simulink model "hovergames"  (R2020b)
settings: Solver=FixedStepAuto  StartTime=0.0  StopTime=20  RelTol=1e-3  EnableMultiTasking=on
undefined symbols (not defined in the file): hovergames_activesm, hovergames_sm
libraries: px4uORBlib x6, dspstat3 x1
settings Model: SimulationMode=external  ExtModeTrigDuration=10  Creator=fabsmpa  LastModifiedBy=fabsmpa
settings SolverCC: PositivePriorityOrder=on
settings OptimizationCC: EnhancedBackFolding=on  PassReuseOutputArgsAs=Individual arguments  ZeroExternalMemoryAtStartup=off  ZeroInternalMemoryAtStartup=off  MaxStackSize=64  OptimizeBlockOrder=speed  DifferentSizesBufferReuse=on  OptimizationCustomize=off  EfficientTunableParamExpr=on
settings DebuggingCC: ParameterTunabilityLossMsg=error
settings HardwareCC: ProdBitPerPointer=32  ProdBitPerSizeT=32  ProdBitPerPtrDiffT=32  ProdLargestAtomicInteger=Long  ProdLargestAtomicFloat=Double  ProdWordSize=32  ProdLongLongMode=on  ProdHWDeviceType=ARM Compatible->ARM Cortex  TargetLargestAtomicInteger=Long  TargetLargestAtomicFloat=Double  TargetIntDivRoundTo=Zero  TargetEndianess=LittleEndian  TargetHWDeviceType=NXP->Cortex-M4
settings SFSimCC: MATLABDynamicMemAlloc=off  SimTargetLang=C++
settings RTWCC: Description=Embedded Coder  SystemTargetFile=ert.tlc  HardwareBoard=PX4 Pixhawk Series  TLCOptions="-aInlineSetEventsForThisBaseRateFcn=TLC_FALSE -aSuppressMultiTaskScheduler=TLC_FALSE  -aRateBasedStepFcn=0"  GenCodeOnly=on  TemplateMakefile=ert_default_tmf  Toolchain=GNU Tools for ARM Embedded Processors  CodeProfilingInstrumentation=detailed  TargetLang=C++
settings CodeAppCC: ForceParamTrailComments=on  IgnoreCustomStorageClasses=off  OperatorAnnotations=on  SimulinkDataObjDesc=on  SFDataObjDesc=on  InsertBlockDesc=on
settings ERTTargetCC: CodeInterfacePackaging=C++ class  RootIOFormat=Structure reference

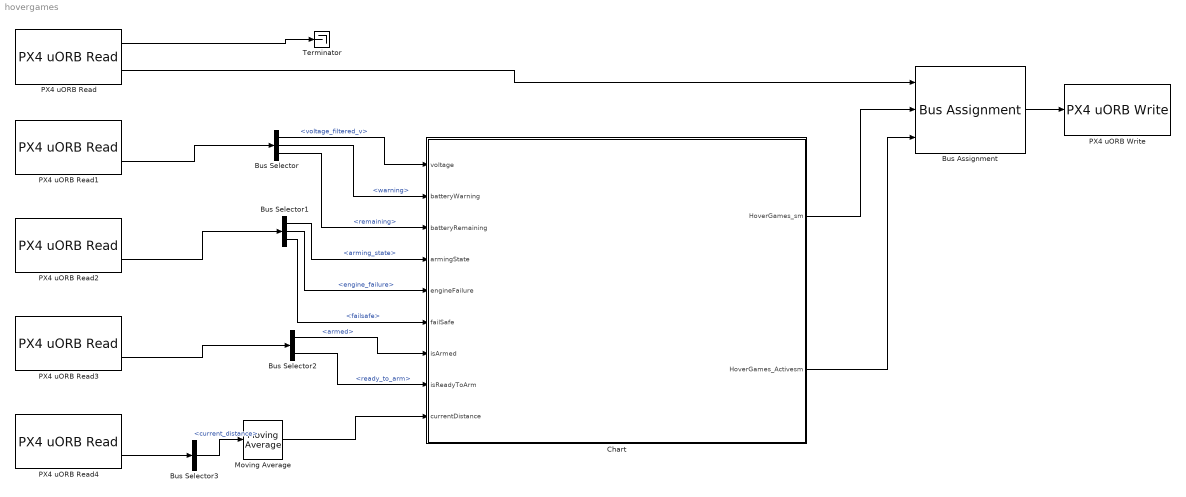
== system hovergames ==
  Bus Assignment : BusAssignment  AssignedSignals=hovergames_sm,hovergames_activesm
  Bus Selector : BusSelector  OutputSignals=voltage_filtered_v,warning,remaining
  Bus Selector1 : BusSelector  OutputSignals=arming_state,engine_failure,failsafe
  Bus Selector2 : BusSelector  OutputSignals=armed,ready_to_arm
  Bus Selector3 : BusSelector  OutputSignals=current_distance
  Chart : Stateflow chart
  Moving Average : dspstat3/Moving Average  Method=Exponential weighting  ForgettingFactorPort=off  SpecifyWindowLength=on  WindowLength=4  ForgettingFactor=0.9  SimulateUsing=Code generation
  PX4 uORB Read : px4uORBlib/PX4 uORB Read  uORBTopic=hovergames  selectInstance=hovergames  SampleTime=0.001  BlockingMode=off  BlockTimeout=1e-3
      settings: SourceProductBaseCode=PX4AUTOPILOTS
  PX4 uORB Read1 : px4uORBlib/PX4 uORB Read  uORBTopic=battery_status  selectInstance=battery_status  SampleTime=0.001  BlockingMode=off  BlockTimeout=1e-3
      settings: SourceProductBaseCode=PX4AUTOPILOTS
  PX4 uORB Read2 : px4uORBlib/PX4 uORB Read  uORBTopic=vehicle_status  selectInstance=vehicle_status  SampleTime=0.001  BlockingMode=off  BlockTimeout=1e-3
      settings: SourceProductBaseCode=PX4AUTOPILOTS
  PX4 uORB Read3 : px4uORBlib/PX4 uORB Read  uORBTopic=actuator_armed  selectInstance=actuator_armed  SampleTime=0.001  BlockingMode=off  BlockTimeout=1e-3
      settings: SourceProductBaseCode=PX4AUTOPILOTS
  PX4 uORB Read4 : px4uORBlib/PX4 uORB Read  uORBTopic=distance_sensor  selectInstance=distance_sensor  SampleTime=0.001  BlockingMode=off  BlockTimeout=1e-3
      settings: SourceProductBaseCode=PX4AUTOPILOTS
  PX4 uORB Write : px4uORBlib/PX4 uORB Write  uORBTopic=hovergames  selectInstance=hovergames  MessageQueueLen=1
      settings: SourceProductBaseCode=PX4AUTOPILOTS
  Terminator : Terminator
  wires:
  PX4 uORB Read/2 -> Bus Assignment/1
  PX4 uORB Read1/2 -> Bus Selector/1
  PX4 uORB Read2/2 -> Bus Selector1/1
  PX4 uORB Read3/2 -> Bus Selector2/1
  PX4 uORB Read4/2 -> Bus Selector3/1
  Bus Selector3/1 -> Moving Average/1  "<current_distance>"
  Bus Selector/1 -> Chart/1(voltage)  "<voltage_filtered_v>"
  Bus Selector/2 -> Chart/2(batteryWarning)  "<warning>"
  Bus Selector/3 -> Chart/3(batteryRemaining)  "<remaining>"
  Bus Selector1/1 -> Chart/4(armingState)  "<arming_state>"
  Bus Selector1/2 -> Chart/5(engineFailure)  "<engine_failure>"
  Bus Selector1/3 -> Chart/6(failSafe)  "<failsafe>"
  Bus Selector2/1 -> Chart/7(isArmed)  "<armed>"
  Bus Selector2/2 -> Chart/8(isReadyToArm)  "<ready_to_arm>"
  Moving Average/1 -> Chart/9(currentDistance)
  Chart/1(HoverGames_sm) -> Bus Assignment/2
  Chart/2(HoverGames_Activesm) -> Bus Assignment/3
  Bus Assignment/1 -> PX4 uORB Write/1
  PX4 uORB Read/1 -> Terminator/1

== stateflow chart hovergames/Chart ==
  state Faulted
    entry:
    HoverGames_sm = FAULTED_STATE;
  state Standby
    entry:
    HoverGames_sm = STANDBY_STATE;
  state Active
    entry:
    HoverGames_sm = ACTIVE_STATE;
    state Recording
      entry:
      HoverGames_Activesm = RECORDING_STATE
    state Paused
      entry:
      HoverGames_Activesm = PAUSED_STATE;
    state ImageCapture
      entry:
      HoverGames_Activesm = IMAGE_CAPTURE_STATE
    (default) -> Paused
    Recording -> Paused [order 1] : [currentDistance <  100 || voltage < 13]
    Paused -> ImageCapture : [currentDistance >= 100]
    ImageCapture -> Paused [order 2] : [currentDistance <  100 || voltage < 13]
    ImageCapture -> Recording [order 1] : [currentDistance >= 1000]
    Recording -> ImageCapture [order 2] : [currentDistance < 1000]
  state PreActive
    entry:
    HoverGames_sm = PREACTIVE_STATE;
  Faulted -> Standby : [engineFailure ==false || batteryWarning == 0 || failSafe == false]
  (default) -> Standby
  Standby -> Faulted [order 2] : [engineFailure == true || batteryWarning > 0 || failSafe == true||  batteryRemaining < 0.4]
  PreActive -> Faulted [order 3] : [engineFailure == true || batteryWarning > 0 || failSafe == true || batteryRemaining < 0.4]
  Active -> Faulted [order 1] : [engineFailure == true || batteryWarning > 0 || failSafe == true || batteryRemaining < 0.4]
  Standby -> PreActive [order 1] : [isReadyToArm==true]
  PreActive -> Standby [order 2] : [isArmed == false]
  Active -> PreActive [order 2] : [isArmed == false]
  PreActive -> Active [order 1] : [isArmed == true && armingState== ARMING_STATE_ARMED]
  data: voltage input single; batteryWarning input uint8; batteryRemaining input; armingState input uint8; engineFailure input boolean; failSafe input boolean; isArmed input boolean; isReadyToArm input boolean; currentDistance input uint32; HoverGames_sm output uint8; HoverGames_Activesm output uint8; STANDBY_STATE constant uint8 =0; PREACTIVE_STATE constant uint8 =1; ACTIVE_STATE constant uint8 =2; FAULTED_STATE constant uint8 =3; RECORDING_STATE constant uint8 =0; IMAGE_CAPTURE_STATE constant uint8 =1; PAUSED_STATE constant uint8 =2; ARMING_STATE_ARMED constant uint8 =2
